simulink model "Spring_Mass_Damper_Model"  (R2018a)
settings: Solver=FixedStepAuto  StartTime=0.0  StopTime=10.0  FixedStep=.0025  RelTol=1e-3
undefined symbols (not defined in the file or in its folder): b, k, m
settings Model: Creator=ameli  LastModifiedBy=ameli

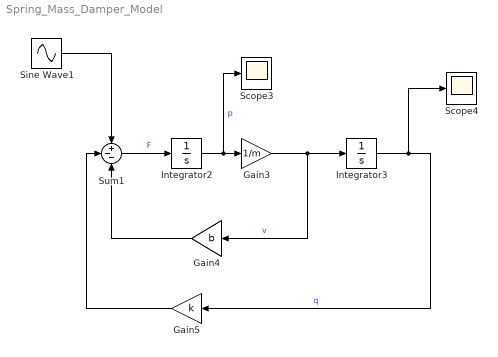
== system Spring_Mass_Damper_Model ==
  Gain3 : Gain  Gain=1/m
  Gain4 : Gain  Gain=b
  Gain5 : Gain  Gain=k
  Integrator2 : Integrator
  Integrator3 : Integrator
  Scope3 : Scope
  Scope4 : Scope
  Sine Wave1 : Sin  Frequency=20*pi  SampleTime=0
  Sum1 : Sum  Inputs=+--
  wires:
  Sine Wave1/1 -> Sum1/1
  Sum1/1 -> Integrator2/1  "F"
  Integrator2/1 -> Scope3/1, Gain3/1  "p"
  Gain3/1 -> Integrator3/1, Gain4/1  "v"
  Integrator3/1 -> Gain5/1, Scope4/1  "q"
  Gain4/1 -> Sum1/3
  Gain5/1 -> Sum1/2
